simulink model "FM_MusicTransmission"  (R2018a)
settings: Solver=VariableStepAuto  StartTime=0.0  StopTime=10.0  RelTol=1e-3
undefined symbols (not defined in the file or in its folder): designMultirateFIR
libraries: dspmlti4 x3, dspfdesign x2, dspsnks4 x1, dspvision x1
settings Model: Creator=Neo  LastModifiedBy=Neo

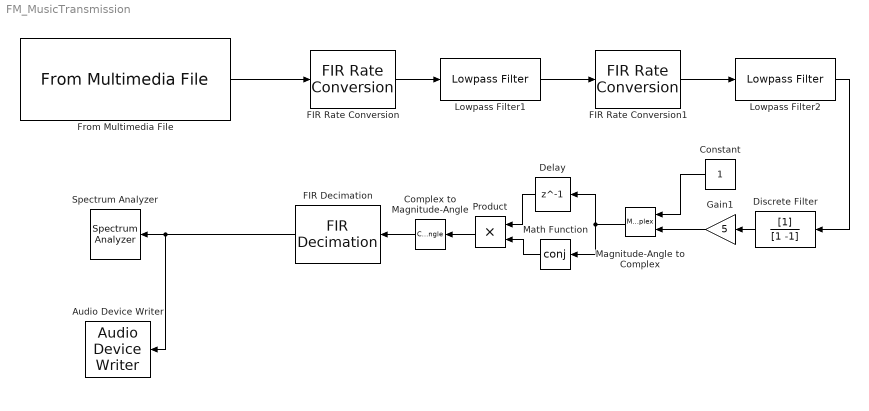
== system FM_MusicTransmission ==
  Audio Device Writer : dspsnks4/Audio Device Writer  Driver=DirectSound  Device=Default  InheritSampleRate=on  SampleRate=44100  BitDepth=16-bit integer  BufferSize=4096  NumBuffers=10  DefaultOutputChannelMapping=on  OutputChannelMapping=1:2  OutputNumUnderrunSamples=off  DriverIdx=1  DeviceWarnFlag=''
  Complex to Magnitude-Angle : ComplexToMagnitudeAngle  Output=Angle
  Constant : Constant
  Delay : Delay  DelayLength=1
  Discrete Filter : DiscreteFilter  Denominator=[1 -1]
  FIR Decimation : dspmlti4/FIR Decimation  FilterSource=Auto  h=designMultirateFIR(1,2)  D=5  filtStruct=Direct form  FilterObject=FDECIM  InputProcessing=Columns as channels (frame based)  framing=Enforce single-rate processing  inputOffset=0  outputBufInitCond=0  roundingMode=Floor  overflowMode=off  firstCoeffDataTypeStr=Inherit: Same word length as input  firstCoeffMin=[]  firstCoeffMax=[]  firstCoeffLastDataTypeStr=Inherit: Same word length as input  outputDataTypeStr=Inherit: Same as accumulator  outputMin=[]  outputMax=[]  outputLastDataTypeStr=Inherit: Same as accumulator
  FIR Rate Conversion : dspmlti4/FIR Rate Conversion  FilterSource=Dialog parameters  L=5  h=firpm(50,[0 15e3 24e3 240e3/2]/(240e3/2),[1 1 0 0],[1 1],20)  M=2  FilterObject=FRC  roundingMode=Floor  overflowMode=off  firstCoeffDataTypeStr=Inherit: Same word length as input  firstCoeffMin=[]  firstCoeffMax=[]  firstCoeffLastDataTypeStr=Inherit: Same word length as input  outputDataTypeStr=Inherit: Same as accumulator  outputMin=[]  outputMax=[]  outputLastDataTypeStr=Inherit: Same as accumulator
      settings: SourceProductName=DSP System Toolbox  SourceProductBaseCode=DS
  FIR Rate Conversion1 : dspmlti4/FIR Rate Conversion  FilterSource=Dialog parameters  L=5  h=firpm(100,[0 15e3 30e3 600e3/2]/(600e3/2),[1 1 0 0],[1 1],20)  M=3  FilterObject=FRC  roundingMode=Floor  overflowMode=off  firstCoeffDataTypeStr=Inherit: Same word length as input  firstCoeffMin=[]  firstCoeffMax=[]  firstCoeffLastDataTypeStr=Inherit: Same word length as input  outputDataTypeStr=Inherit: Same as accumulator  outputMin=[]  outputMax=[]  outputLastDataTypeStr=Inherit: Same as accumulator
      settings: SourceProductName=DSP System Toolbox  SourceProductBaseCode=DS
  From Multimedia File : dspvision/From Multimedia File  inputFilename=D:\KTÜ Dersleri\3-2\İletişim Tekniği\Laboratuvar\1\piano.mp3  loop=on  numPlays=inf  outputStreams=Audio only  videoDataType=single  audioDataType=double  inheritSampleTime=on  userDefinedSampleTime=1/30  noAudioOutput=off  isIntensityVideo=off  fourcc=RGB  colorVideoFormat=Separate color signals  outputEOF=off  dataOrg=Column-major  audioFrameSize=48000  computeAudioFrameSize=off  outSamplingMode=Sample based
      settings: SourceProductBaseCode=VP
  Gain1 : Gain  Gain=5
  Lowpass Filter1 : dspfdesign/Lowpass Filter  FilterType=FIR  DesignForMinimumOrder=off  FilterOrder=100  PassbandFrequency=15e3  StopbandFrequency=12e3  PassbandRipple=0.1  StopbandAttenuation=80  InheritSampleRate=off  SampleRate=120e3  SimulateUsing=Interpreted execution  roundingMode=Floor  coeffsDataTypeStr=fixdt(1,16)
  Lowpass Filter2 : dspfdesign/Lowpass Filter  FilterType=FIR  DesignForMinimumOrder=off  FilterOrder=100  PassbandFrequency=15e3  StopbandFrequency=12e3  PassbandRipple=0.1  StopbandAttenuation=80  InheritSampleRate=off  SampleRate=200e3  SimulateUsing=Interpreted execution  roundingMode=Floor  coeffsDataTypeStr=fixdt(1,16)
  Magnitude-Angle to Complex : MagnitudeAngleToComplex
  Math Function : Math  Operator=conj  SaturateOnIntegerOverflow=on
  Product : Product
  Spectrum Analyzer : SpectrumAnalyzer
  wires:
  From Multimedia File/1 -> FIR Rate Conversion/1
  FIR Rate Conversion/1 -> Lowpass Filter1/1
  Lowpass Filter1/1 -> FIR Rate Conversion1/1
  FIR Rate Conversion1/1 -> Lowpass Filter2/1
  Gain1/1 -> Magnitude-Angle to Complex/2
  Constant/1 -> Magnitude-Angle to Complex/1
  Discrete Filter/1 -> Gain1/1
  Lowpass Filter2/1 -> Discrete Filter/1
  Math Function/1 -> Product/2
  Delay/1 -> Product/1
  Product/1 -> Complex to Magnitude-Angle/1
  Magnitude-Angle to Complex/1 -> Delay/1, Math Function/1
  Complex to Magnitude-Angle/1 -> FIR Decimation/1
  FIR Decimation/1 -> Audio Device Writer/1, Spectrum Analyzer/1
